simulink model "mass"  (R2016a)
settings: Solver=VariableStepAuto  StartTime=0.0  StopTime=10.0  RelTol=1e-3
undefined symbols (not defined in the file): b, k, m
settings Model: Creator=Islam Barakat  LastModifiedBy=Islam Barakat
settings OptimizationCC: BlockReduction=off  DefaultParameterBehavior=Inlined  BufferReuse=off

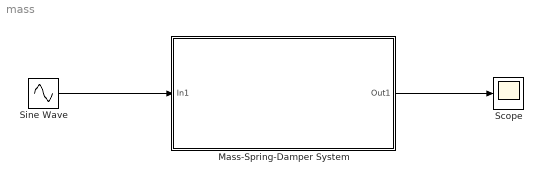
== system mass ==
  Mass-Spring-Damper System : Subsystem
      mask Display:
      | set_param(gcbh, 'BackgroundColor','Orange');
      | disp('Mass-Spring-Damper System');
  Scope : Scope
  Sine Wave : Sin  Amplitude=12  Bias=5  Frequency=0.7  Phase=pi  SampleTime=0
  wires:
  Sine Wave/1 -> Mass-Spring-Damper System/1(In1)
  Mass-Spring-Damper System/1(Out1) -> Scope/1

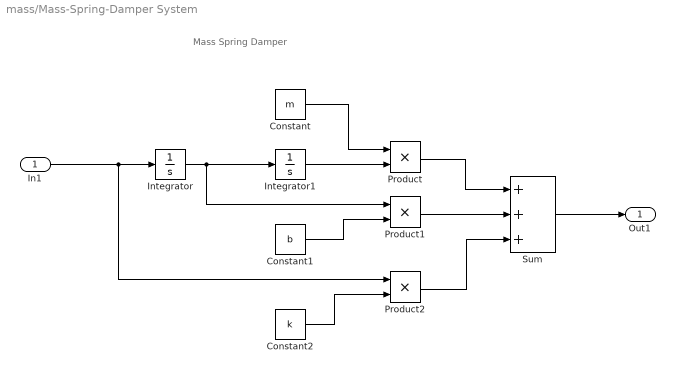
== system mass/Mass-Spring-Damper System ==
  note: Mass Spring Damper
  In1 : Inport
  Constant : Constant  Value=m
      mask Display:
      | set_param(get_param(gcb,'Handle'),'BackgroundColor','Cyan');
      | disp('Mass');
  Constant1 : Constant  Value=b
      mask Display:
      | set_param(get_param(gcb,'Handle'),'BackgroundColor','Yellow');
      | disp('Damp');
  Constant2 : Constant  Value=k
      mask Display:
      | set_param(get_param(gcb,'Handle'),'BackgroundColor','Green');
      | disp('Spring');
  Integrator : Integrator
  Integrator1 : Integrator
  Product : Product
  Product1 : Product
  Product2 : Product
  Sum : Sum  Inputs=+++
  Out1 : Outport
  wires:
  Product2/1 -> Sum/3
  Constant/1 -> Product/1
  Integrator/1 -> Product1/1, Integrator1/1
  Product/1 -> Sum/1
  Constant2/1 -> Product2/2
  Constant1/1 -> Product1/2
  Integrator1/1 -> Product/2
  Product1/1 -> Sum/2
  In1/1 -> Product2/1, Integrator/1
  Sum/1 -> Out1/1
